simulink model "ASM_Traffic_V2X_Complete_Model_2"  (R2019a)
settings: Solver=ode1  StartTime=SIM.tstart.v  StopTime=Inf  FixedStep=SIM.StepSize.v  RelTol=1e-3
PostLoadFcn:
  | if any(exist('dsrtsu_mdlpostloadfcn', 'file') ~= 0), dsrtsu_mdlpostloadfcn('Execute', bdroot); end
  | try, asm_mdl_postloadfcn(bdroot, 'UpdateModel', 2200); catch, disp(lasterr); end,
undefined symbols (not defined in the file): _SensorPnts_1, _SensorPnts_13, _SensorPnts_17, _SensorPnts_21, _SensorPnts_25, _SensorPnts_29, _SensorPnts_33, _SensorPnts_37, _SensorPnts_41, _SensorPnts_45, _SensorPnts_49, _SensorPnts_5, _SensorPnts_53, _SensorPnts_57, _SensorPnts_9, _to_, CPT, G5A, ITS, MDL, rad, s_to_rpm, SIM
libraries: simulink x169, ASM_VehicleDynamics_lib x126, ASM_Traffic_lib x83, ASM_Utils_lib x49, mdbs x45, ASM_Environment_lib x17, dspindex x12, dsaV2xLibraryAux x10, dsmpblib x6, dsaV2xAsn1Library x4, dsaV2xLibrary x4, ASM_BrakeHydraulics_lib x4
(part 24 of 36)

== system ASM_Traffic_V2X_Complete_Model_2/MDL/Environment/EnvironmentInterface_In/VehicleMovement/Mapping_Vel/YawRate_Vehicle_CoG[deg|s]1 ==
  In1 : Inport
  Out1 : Outport
  wires:
  In1/1 -> Out1/1

== system ASM_Traffic_V2X_Complete_Model_2/MDL/Environment/EnvironmentInterface_In/VehicleMovement/Mapping_Vel/v_x_Vehicle_CoG[km|h]1 ==
  In1 : Inport
  Out1 : Outport
  wires:
  In1/1 -> Out1/1

== system ASM_Traffic_V2X_Complete_Model_2/MDL/Environment/EnvironmentInterface_In/VehicleMovement/Mapping_Vel/v_y_Vehicle_CoG[km|h]1 ==
  In1 : Inport
  Out1 : Outport
  wires:
  In1/1 -> Out1/1

== system ASM_Traffic_V2X_Complete_Model_2/MDL/Environment/Maneuver/ExternalSegmentEnd/Dist_Front_Min/Replace_NoObjectFound1 ==
  In1 : Inport
  Far_away : Constant  Value=1000
  No_Hinderance : Constant  Value=0
  Relational Operator : RelationalOperator  Operator=<=  RndMeth=Nearest  InputSameDT=on
  Switch : Switch  Threshold=1  InputSameDT=on
  Out1 : Outport
  wires:
  No_Hinderance/1 -> Relational Operator/2
  Relational Operator/1 -> Switch/2
  Far_away/1 -> Switch/1
  In1/1 -> Relational Operator/1, Switch/3
  Switch/1 -> Out1/1

== system ASM_Traffic_V2X_Complete_Model_2/MDL/Environment/Maneuver/ExternalSegmentEnd/Dist_Rear_Min/Replace_NoObjectFound1 ==
  In1 : Inport
  Far_away : Constant  Value=1000
  No_Hinderance : Constant  Value=0
  Relational Operator : RelationalOperator  Operator=<=  RndMeth=Nearest  InputSameDT=on
  Switch : Switch  Threshold=1  InputSameDT=on
  Out1 : Outport
  wires:
  Switch/1 -> Out1/1
  In1/1 -> Switch/3, Relational Operator/1
  Far_away/1 -> Switch/1
  Relational Operator/1 -> Switch/2
  No_Hinderance/1 -> Relational Operator/2

== system ASM_Traffic_V2X_Complete_Model_2/MDL/Environment/Maneuver/ExternalSegmentEnd/SegmentEndTrigger/Fishhook ==
  RollRate_Threshold[deg|s] : Inport
  RollRate_Vehicle_CoG[deg|s] : Inport  Port=2
  Abs : Abs  SaturateOnIntegerOverflow=on
  Fcn_1 : Fcn  Expr=(u[1]>=0.0)*(u[2]<0.0)
  Fcn_2 : Fcn  Expr=(u[1]>0.0)
  Memory1 : Memory
  Memory2 : Memory
  Mux : Mux  Inputs=2
  Product : Product  RndMeth=Zero
  Sum : Sum  Inputs=|-+  SaturateOnIntegerOverflow=on
  SegmentEnd_Fishhook : Outport
  wires:
  Memory1/1 -> Mux/1
  Mux/1 -> Fcn_1/1
  Sum/1 -> Memory1/1, Mux/2
  Abs/1 -> Sum/2
  RollRate_Threshold[deg|s]/1 -> Sum/1, Memory2/1
  RollRate_Vehicle_CoG[deg|s]/1 -> Abs/1
  Memory2/1 -> Fcn_2/1
  Fcn_2/1 -> Product/1
  Fcn_1/1 -> Product/2
  Product/1 -> SegmentEnd_Fishhook/1

== system ASM_Traffic_V2X_Complete_Model_2/MDL/Environment/Maneuver/ExternalSegmentEnd/SegmentEndTrigger/SaturateAndRound ==
  In : Inport
  Max : Inport  Port=2
  Const_zero : Constant  Value=0
  Data Type Conversion : DataTypeConversion
  Log_and : Logic  Inputs=3  AllPortsSameDT=off  OutDataTypeStr=boolean
  Product : Product  RndMeth=Zero
  RelOp1 : RelationalOperator  Operator===  OutDataTypeStr=boolean  RndMeth=Nearest
  RelOp2 : RelationalOperator  Operator=<=  OutDataTypeStr=boolean  RndMeth=Nearest
  RelOp3 : RelationalOperator  OutDataTypeStr=boolean  RndMeth=Nearest
  Round : Rounding  Operator=round
  ExternalSegmentEnd_Mode[] : Outport
  wires:
  In/1 -> Product/1, RelOp2/1, RelOp3/1, RelOp1/2, Round/1
  Round/1 -> RelOp1/1
  RelOp1/1 -> Log_and/1
  Log_and/1 -> Data Type Conversion/1
  Data Type Conversion/1 -> Product/2
  Const_zero/1 -> RelOp3/2
  RelOp3/1 -> Log_and/2
  RelOp2/1 -> Log_and/3
  Product/1 -> ExternalSegmentEnd_Mode[]/1
  Max/1 -> RelOp2/2

== system ASM_Traffic_V2X_Complete_Model_2/MDL/Environment/Traffic/FellowMovement/Customize_UserSignals/Label ==
  In1 : Inport
  Out1 : Outport
  wires:
  In1/1 -> Out1/1

== system ASM_Traffic_V2X_Complete_Model_2/MDL/Environment/Traffic/FellowMovement/Customize_UserSignals/Label1 ==
  In1 : Inport
  Out1 : Outport
  wires:
  In1/1 -> Out1/1

== system ASM_Traffic_V2X_Complete_Model_2/MDL/Environment/Traffic/FellowMovement/Customize_UserSignals/Label10 ==
  In1 : Inport
  Out1 : Outport
  wires:
  In1/1 -> Out1/1

== system ASM_Traffic_V2X_Complete_Model_2/MDL/Environment/Traffic/FellowMovement/Customize_UserSignals/Label11 ==
  In1 : Inport
  Out1 : Outport
  wires:
  In1/1 -> Out1/1

== system ASM_Traffic_V2X_Complete_Model_2/MDL/Environment/Traffic/FellowMovement/Customize_UserSignals/Label12 ==
  In1 : Inport
  Out1 : Outport
  wires:
  In1/1 -> Out1/1

== system ASM_Traffic_V2X_Complete_Model_2/MDL/Environment/Traffic/FellowMovement/Customize_UserSignals/Label13 ==
  In1 : Inport
  Out1 : Outport
  wires:
  In1/1 -> Out1/1

== system ASM_Traffic_V2X_Complete_Model_2/MDL/Environment/Traffic/FellowMovement/Customize_UserSignals/Label14 ==
  In1 : Inport
  Out1 : Outport
  wires:
  In1/1 -> Out1/1

== system ASM_Traffic_V2X_Complete_Model_2/MDL/Environment/Traffic/FellowMovement/Customize_UserSignals/Label2 ==
  In1 : Inport
  Out1 : Outport
  wires:
  In1/1 -> Out1/1

== system ASM_Traffic_V2X_Complete_Model_2/MDL/Environment/Traffic/FellowMovement/Customize_UserSignals/Label3 ==
  In1 : Inport
  Out1 : Outport
  wires:
  In1/1 -> Out1/1

== system ASM_Traffic_V2X_Complete_Model_2/MDL/Environment/Traffic/FellowMovement/Customize_UserSignals/Label4 ==
  In1 : Inport
  Out1 : Outport
  wires:
  In1/1 -> Out1/1

== system ASM_Traffic_V2X_Complete_Model_2/MDL/Environment/Traffic/FellowMovement/Customize_UserSignals/Label5 ==
  In1 : Inport
  Out1 : Outport
  wires:
  In1/1 -> Out1/1

== system ASM_Traffic_V2X_Complete_Model_2/MDL/Environment/Traffic/FellowMovement/Customize_UserSignals/Label6 ==
  In1 : Inport
  Out1 : Outport
  wires:
  In1/1 -> Out1/1

== system ASM_Traffic_V2X_Complete_Model_2/MDL/Environment/Traffic/FellowMovement/Customize_UserSignals/Label7 ==
  In1 : Inport
  Out1 : Outport
  wires:
  In1/1 -> Out1/1

== system ASM_Traffic_V2X_Complete_Model_2/MDL/Environment/Traffic/FellowMovement/Customize_UserSignals/Label8 ==
  In1 : Inport
  Out1 : Outport
  wires:
  In1/1 -> Out1/1

== system ASM_Traffic_V2X_Complete_Model_2/MDL/Environment/Traffic/FellowMovement/Customize_UserSignals/Label9 ==
  In1 : Inport
  Out1 : Outport
  wires:
  In1/1 -> Out1/1

== system ASM_Traffic_V2X_Complete_Model_2/MDL/Environment/Traffic/FellowMovement/LabelUserSignals/UserSignals_ ==
  UserSignals : Inport
  Demux : Demux  Outputs=5
  User1[] : Outport
  User2[] : Outport  Port=2
  User3[] : Outport  Port=3
  User4[] : Outport  Port=4
  User5[] : Outport  Port=5
  wires:
  Demux/5 -> User5[]/1
  Demux/4 -> User4[]/1
  UserSignals/1 -> Demux/1
  Demux/1 -> User1[]/1
  Demux/2 -> User2[]/1
  Demux/3 -> User3[]/1

== system ASM_Traffic_V2X_Complete_Model_2/MDL/Environment/Traffic/FellowMovement/LabelUserSignals_Fellows/UserSignals_ ==
  UserSignals : Inport
  Demux : Demux  Outputs=15
  UserSignals_Fellow1[] : Outport
  UserSignals_Fellow2[] : Outport  Port=2
  UserSignals_Fellow3[] : Outport  Port=3
  UserSignals_Fellow4[] : Outport  Port=4
  UserSignals_Fellow5[] : Outport  Port=5
  UserSignals_Fellow6[] : Outport  Port=6
  UserSignals_Fellow7[] : Outport  Port=7
  UserSignals_Fellow8[] : Outport  Port=8
  UserSignals_Fellow9[] : Outport  Port=9
  UserSignals_Fellow10[] : Outport  Port=10
  UserSignals_Fellow11[] : Outport  Port=11
  UserSignals_Fellow12[] : Outport  Port=12
  UserSignals_Fellow13[] : Outport  Port=13
  UserSignals_Fellow14[] : Outport  Port=14
  UserSignals_Fellow15[] : Outport  Port=15
  wires:
  Demux/15 -> UserSignals_Fellow15[]/1  "User1[]"
  Demux/14 -> UserSignals_Fellow14[]/1  "User2[]"
  Demux/13 -> UserSignals_Fellow13[]/1  "User1[]"
  Demux/12 -> UserSignals_Fellow12[]/1  "User2[]"
  Demux/11 -> UserSignals_Fellow11[]/1  "User1[]"
  Demux/10 -> UserSignals_Fellow10[]/1  "User2[]"
  Demux/9 -> UserSignals_Fellow9[]/1  "User1[]"
  Demux/8 -> UserSignals_Fellow8[]/1  "User2[]"
  Demux/7 -> UserSignals_Fellow7[]/1  "User1[]"
  Demux/6 -> UserSignals_Fellow6[]/1  "User2[]"
  Demux/5 -> UserSignals_Fellow5[]/1  "User1[]"
  Demux/4 -> UserSignals_Fellow4[]/1  "User2[]"
  Demux/3 -> UserSignals_Fellow3[]/1  "User1[]"
  Demux/2 -> UserSignals_Fellow2[]/1  "User2[]"
  Demux/1 -> UserSignals_Fellow1[]/1  "User1[]"
  UserSignals/1 -> Demux/1

== system ASM_Traffic_V2X_Complete_Model_2/MDL/Environment/Traffic/FellowMovement/Sw_SpeedLimit_Enable/SpeedLimit_RateLimiter ==
  In : Inport
  Gain : Gain  Gain=-1
  Multiport Switch : MultiPortSwitch  DataPortOrder=Zero-based contiguous  Inputs=2  DiagnosticForDefault=Warning  zeroidx=on
  Rate Limiter Dynamic : simulink/Discontinuities/Rate Limiter Dynamic
      settings: SourceProductName=Simulink
  RateLimit_ActivateThreshold[km|h] : simulink/Logic and Bit Operations/Compare To Constant  relop=>  const=200  OutDataTypeStr=uint8
  SpeedLimit_ChangeRate[km|h|s] : Constant  Value=20.0*ones(MDL.Traffic.MaxNumFellows.v,1)
  Unit Delay : UnitDelay  SampleTime=-1
  off : Constant  Value=1e8*ones(MDL.Traffic.MaxNumFellows.v,1)
  Out : Outport
  wires:
  Unit Delay/1 -> Rate Limiter Dynamic/1, Gain/1
  Rate Limiter Dynamic/1 -> Out/1
  In/1 -> RateLimit_ActivateThreshold[km|h]/1, Rate Limiter Dynamic/2
  Gain/1 -> Rate Limiter Dynamic/3
  Multiport Switch/1 -> Unit Delay/1
  SpeedLimit_ChangeRate[km|h|s]/1 -> Multiport Switch/2
  off/1 -> Multiport Switch/3
  RateLimit_ActivateThreshold[km|h]/1 -> Multiport Switch/1

== system ASM_Traffic_V2X_Complete_Model_2/MDL/Environment/Traffic/Sensors/Collision_Sensor/ASMSignalCollector ==
  Bus Creator3 : BusCreator  Inputs=1
  tag scope: ASMBUS_Environment_Traffic_Sensors_Collision_Sensor=global
  wires:
  [ASMBUS_Traf_Sensors_Collision_Sensor_1] -> Bus Creator3/1  "Collision_Sensor_1"
  Bus Creator3/1 -> [ASMBUS_Environment_Traffic_Sensors_Collision_Sensor]  "Collision_Sensor"

== system ASM_Traffic_V2X_Complete_Model_2/MDL/Environment/Traffic/Sensors/Collision_Sensor/Enable_Collision_Sensor ==
  Enable_In[0Off|1On] : Inport
  Constant : Constant  Value=0.5  SampleTime=-1
  Constant1 : Constant  SampleTime=-1
  Constant2 : Constant  Value=0  SampleTime=-1
  Enable_Sensor : Gain
  Multiport Switch : MultiPortSwitch  DataPortOrder=Zero-based contiguous  Inputs=2  zeroidx=on
  Relational Operator : RelationalOperator  Operator=>  OutDataTypeStr=boolean  RndMeth=Nearest
  Enable_Out[0Off|1On] : Outport
  wires:
  Enable_In[0Off|1On]/1 -> Enable_Sensor/1
  Enable_Sensor/1 -> Relational Operator/1
  Relational Operator/1 -> Multiport Switch/1
  Multiport Switch/1 -> Enable_Out[0Off|1On]/1
  Constant/1 -> Relational Operator/2
  Constant1/1 -> Multiport Switch/3
  Constant2/1 -> Multiport Switch/2

== system ASM_Traffic_V2X_Complete_Model_2/MDL/Environment/Traffic/Sensors/Custom_Sensor/ASMSignalBus_Mapping ==
  ScopezoneData : Inport
  ObjectData : Inport  Port=2
  Bus Creator : BusCreator  Inputs=5
  Bus Creator1 : BusCreator  Inputs=2
  Bus Selector6 : BusSelector  OutputSignals=Info,SensorOutput.Object1,SensorOutput.Object2,SensorOutput.Object3,SensorOutput.Object4,SensorOutput.Object5
  Bus Selector8 : BusSelector  OutputSignals=Info,SensorOutput.Object1,SensorOutput.Object2,SensorOutput.Object3,SensorOutput.Object4,SensorOutput.Object5
  Combine1 : Subsystem
  Combine2 : Subsystem
  Combine3 : Subsystem
  Combine4 : Subsystem
  Combine5 : Subsystem
  CombineInfo : Subsystem
  ASMSignalBus : Outport
  wires:
  CombineInfo/1(Combined_Out) -> Bus Creator1/1  "Info"
  Bus Selector8/1 -> CombineInfo/2(Values_In)  "<Info>"
  Bus Selector6/1 -> CombineInfo/1(Scopezone_In)  "<Info>"
  Bus Creator1/1 -> ASMSignalBus/1
  Bus Selector6/2 -> Combine1/1(Scopezone_In)  "<Object1>"
  Bus Selector8/2 -> Combine1/2(Values_In)  "<Object1>"
  ScopezoneData/1 -> Bus Selector6/1
  ObjectData/1 -> Bus Selector8/1
  Combine1/1(Combined_Out) -> Bus Creator/1  "Object1"
  Combine2/1(Combined_Out) -> Bus Creator/2  "Object2"
  Bus Selector6/3 -> Combine2/1(Scopezone_In)  "<Object2>"
  Bus Selector8/3 -> Combine2/2(Values_In)  "<Object2>"
  Combine3/1(Combined_Out) -> Bus Creator/3  "Object3"
  Bus Selector6/4 -> Combine3/1(Scopezone_In)  "<Object3>"
  Bus Selector8/4 -> Combine3/2(Values_In)  "<Object3>"
  Combine4/1(Combined_Out) -> Bus Creator/4  "Object4"
  Bus Selector6/5 -> Combine4/1(Scopezone_In)  "<Object4>"
  Bus Selector8/5 -> Combine4/2(Values_In)  "<Object4>"
  Combine5/1(Combined_Out) -> Bus Creator/5  "Object5"
  Bus Selector8/6 -> Combine5/2(Values_In)  "<Object5>"
  Bus Selector6/6 -> Combine5/1(Scopezone_In)  "<Object5>"
  Bus Creator/1 -> Bus Creator1/2  "SensorOutput"

== system ASM_Traffic_V2X_Complete_Model_2/MDL/Environment/Traffic/Sensors/Custom_Sensor/ASMSignalCollector ==
  Bus Creator1 : BusCreator  Inputs=3
  Bus Creator3 : BusCreator  Inputs=1
  Bus Selector : BusSelector  OutputSignals=Info,SensorOutput
  tag scope: ASMBUS_Environment_Traffic_Sensors_Custom_Sensor=global
  wires:
  [ASMBUS_Environment_Traffic_Sensors_Custom_Sensor_1_Parameters] -> Bus Creator1/3  "Parameters"
  Bus Selector/2 -> Bus Creator1/2  "<SensorOutput>"
  Bus Selector/1 -> Bus Creator1/1  "<Info>"
  [ASMBUS_Environment_Traffic_Sensors_Custom_Sensor_1] -> Bus Selector/1
  Bus Creator3/1 -> [ASMBUS_Environment_Traffic_Sensors_Custom_Sensor]  "Custom_Sensor"
  Bus Creator1/1 -> Bus Creator3/1  "Sensor_Front_1"

== system ASM_Traffic_V2X_Complete_Model_2/MDL/Environment/Traffic/Sensors/Custom_Sensor/Enable_Custom_Sensor ==
  Enable_In[0Off|1On] : Inport
  Constant : Constant  Value=0.5  SampleTime=-1
  Constant1 : Constant  SampleTime=-1
  Constant2 : Constant  Value=0  SampleTime=-1
  Enable_Sensor : Gain
  Multiport Switch : MultiPortSwitch  DataPortOrder=Zero-based contiguous  Inputs=2  zeroidx=on
  Relational Operator : RelationalOperator  Operator=>  OutDataTypeStr=boolean  RndMeth=Nearest
  Enable_Out[0Off|1On] : Outport
  wires:
  Constant2/1 -> Multiport Switch/2
  Constant1/1 -> Multiport Switch/3
  Constant/1 -> Relational Operator/2
  Multiport Switch/1 -> Enable_Out[0Off|1On]/1
  Relational Operator/1 -> Multiport Switch/1
  Enable_Sensor/1 -> Relational Operator/1
  Enable_In[0Off|1On]/1 -> Enable_Sensor/1

== system ASM_Traffic_V2X_Complete_Model_2/MDL/Environment/Traffic/Sensors/Custom_Sensor/SensorOutput_Mapping ==
  ScopezoneData : Inport
  ObjectData : Inport  Port=2
  Bus Creator : BusCreator  Inputs=5
  Bus Creator1 : BusCreator  Inputs=1
  Bus Selector6 : BusSelector  OutputSignals=SensorOutput.Object1,SensorOutput.Object2,SensorOutput.Object3,SensorOutput.Object4,SensorOutput.Object5
  Bus Selector8 : BusSelector  OutputSignals=SensorOutput.Object1,SensorOutput.Object2,SensorOutput.Object3,SensorOutput.Object4,SensorOutput.Object5
  Combine1 : Subsystem
  Combine2 : Subsystem
  Combine3 : Subsystem
  Combine4 : Subsystem
  Combine5 : Subsystem
  Sensor_Signals : Outport
  wires:
  Bus Creator/1 -> Bus Creator1/1  "SensorOutput"
  Bus Selector6/5 -> Combine5/1(Scopezone_In)  "<Object5>"
  Bus Selector8/5 -> Combine5/2(Values_In)  "<Object5>"
  Combine5/1(Combined_Out) -> Bus Creator/5  "Object5"
  Bus Selector8/4 -> Combine4/2(Values_In)  "<Object4>"
  Bus Selector6/4 -> Combine4/1(Scopezone_In)  "<Object4>"
  Combine4/1(Combined_Out) -> Bus Creator/4  "Object4"
  Bus Selector8/3 -> Combine3/2(Values_In)  "<Object3>"
  Bus Selector6/3 -> Combine3/1(Scopezone_In)  "<Object3>"
  Combine3/1(Combined_Out) -> Bus Creator/3  "Object3"
  Bus Selector8/2 -> Combine2/2(Values_In)  "<Object2>"
  Bus Selector6/2 -> Combine2/1(Scopezone_In)  "<Object2>"
  Combine2/1(Combined_Out) -> Bus Creator/2  "Object2"
  Combine1/1(Combined_Out) -> Bus Creator/1  "Object1"
  ObjectData/1 -> Bus Selector8/1
  ScopezoneData/1 -> Bus Selector6/1
  Bus Selector8/1 -> Combine1/2(Values_In)  "<Object1>"
  Bus Selector6/1 -> Combine1/1(Scopezone_In)  "<Object1>"
  Bus Creator1/1 -> Sensor_Signals/1

== system ASM_Traffic_V2X_Complete_Model_2/MDL/Environment/Traffic/Sensors/Custom_Sensor/TrafficObject_Type ==
  In1 : Inport
  Bus Selector1 : BusSelector  OutputSignals=SensorOutput.Object1.Object_Type[],SensorOutput.Object2.Object_Type[],SensorOutput.Object3.Object_Type[],SensorOutput.Object4.Object_Type[],SensorOutput.Object5.Object_Type[]
  Mux : Mux  Inputs=5
  Out1 : Outport
  wires:
  Mux/1 -> Out1/1
  Bus Selector1/5 -> Mux/5  "<Object_Type[]>"
  Bus Selector1/4 -> Mux/4  "<Object_Type[]>"
  Bus Selector1/3 -> Mux/3  "<Object_Type[]>"
  Bus Selector1/2 -> Mux/2  "<Object_Type[]>"
  Bus Selector1/1 -> Mux/1  "<Object_Type[]>"
  In1/1 -> Bus Selector1/1

== system ASM_Traffic_V2X_Complete_Model_2/MDL/Environment/Traffic/Sensors/Line_Sensor/ASMSignalCollector ==
  note: LineSensor-Output not
      | fed into SignalBus due
      | to large amount of signal data.
  Add{,1..5} (6 alike) : Sum
  Bus Creator1 : BusCreator  Inputs=8
  Bus Creator{2,4..8} (6 alike) : BusCreator  Inputs=3
  Bus Creator3 : BusCreator  Inputs=1
  Bus Selector : BusSelector  OutputSignals=SensorOutput.Info,SensorOutput.Road,SensorOutput.Junction
  Bus Selector1 : BusSelector  OutputSignals=Road_Lanes.Pos_x_Road_Lanes_CoorSys_E[m],Road_Lanes.Pos_y_Road_Lanes_CoorSys_E[m],Road_Lanes.Pos_z_Road_Lanes_CoorSys_E[m]
  Bus Selector2 : BusSelector  OutputSignals=Junction_Borders.Pos_x_Junction_Borders_CoorSys_E[m],Junction_Borders.Pos_y_Junction_Borders_CoorSys_E[m],Junction_Borders.Pos_z_Junction_Borders_CoorSys_E[m]
  Bus Selector3 : BusSelector  OutputSignals=Road_Shape_Lines.Pos_x_Road_Shape_Lines_CoorSys_E[m],Road_Shape_Lines.Pos_y_Road_Shape_Lines_CoorSys_E[m],Road_Shape_Lines.Pos_z_Road_Shape_Lines_CoorSys_E[m]
  Bus Selector4 : BusSelector  OutputSignals=Road_Shape_ContObj.Pos_x_Road_Shape_ContObj_CoorSys_E[m],Road_Shape_ContObj.Pos_y_Road_Shape_ContObj_CoorSys_E[m],Road_Shape_ContObj.Pos_z_Road_Shape_ContObj_CoorSys_E[m]
  Bus Selector5 : BusSelector  OutputSignals=Junction_Shape_Lines.Pos_x_Junction_Shape_Lines_CoorSys_E[m],Junction_Shape_Lines.Pos_y_Junction_Shape_Lines_CoorSys_E[m],Junction_Shape_Lines.Pos_z_Junction_Shape_Lines_CoorSys_E[m]
  Bus Selector6 : BusSelector  OutputSignals=Junction_Shape_ContObj.Pos_x_Junction_Shape_ContObj_CoorSys_E[m],Junction_Shape_ContObj.Pos_y_Junction_Shape_ContObj_CoorSys_E[m],Junction_Shape_ContObj.Pos_z_Junction_Shape_ContObj_CoorSys_E[m]
  Dummy : Constant  Value=0
  Idx_Vector_Junction_Borders : Constant  Value=1:1:60
  Idx_Vector_Junction_Shape_ContObj : Constant  Value=1:1:60
  Idx_Vector_Junction_Shape_Lines : Constant  Value=1:1:60
  Idx_Vector_Road_Lanes : Constant  Value=1:1:60
  Idx_Vector_Road_Shape_ContObj : Constant  Value=1:1:60
  Idx_Vector_Road_Shape_Lines : Constant  Value=1:1:60
  Saturation : Saturate  UpperLimit=MDL.Traffic.Sensors.LineSensor.Const_Road_Lane_Output_Dimension.v  LowerLimit=1
  Saturation1 : Saturate  UpperLimit=MDL.Traffic.Sensors.LineSensor.Const_Road_Shape_Line_Output_Dimension.v  LowerLimit=1
  Saturation2 : Saturate  UpperLimit=MDL.Traffic.Sensors.LineSensor.Const_Road_Shape_ContObj_Output_Dimension.v  LowerLimit=1
  Saturation3 : Saturate  UpperLimit=MDL.Traffic.Sensors.LineSensor.Const_Junction_Border_Output_Dimension.v  LowerLimit=1
  Saturation4 : Saturate  UpperLimit=MDL.Traffic.Sensors.LineSensor.Const_Junction_Border_Output_Dimension.v  LowerLimit=1
  Saturation5 : Saturate  UpperLimit=MDL.Traffic.Sensors.LineSensor.Const_Junction_Border_Output_Dimension.v  LowerLimit=1
  Selector1 : Selector  InputPortWidth=MDL.Traffic.Sensors.LineSensor.Const_Road_Lane_Output_Dimension.v  IndexOptions=Index vector (port)  Indices=1  OutputSizes=36
  Selector10 : Selector  InputPortWidth=MDL.Traffic.Sensors.LineSensor.Const_Road_Shape_ContObj_Output_Dimension.v  IndexOptions=Index vector (port)  Indices=1  OutputSizes=36
  Selector11 : Selector  InputPortWidth=MDL.Traffic.Sensors.LineSensor.Const_Road_Shape_ContObj_Output_Dimension.v  IndexOptions=Index vector (port)  Indices=1  OutputSizes=36
  Selector12 : Selector  InputPortWidth=MDL.Traffic.Sensors.LineSensor.Const_Road_Shape_ContObj_Output_Dimension.v  IndexOptions=Index vector (port)  Indices=1  OutputSizes=36
  Selector13 : Selector  InputPortWidth=MDL.Traffic.Sensors.LineSensor.Const_Junction_Shape_Line_Output_Dimension.v  IndexOptions=Index vector (port)  Indices=1  OutputSizes=36
  Selector14 : Selector  InputPortWidth=MDL.Traffic.Sensors.LineSensor.Const_Junction_Shape_Line_Output_Dimension.v  IndexOptions=Index vector (port)  Indices=1  OutputSizes=36
  Selector15 : Selector  InputPortWidth=MDL.Traffic.Sensors.LineSensor.Const_Junction_Shape_Line_Output_Dimension.v  IndexOptions=Index vector (port)  Indices=1  OutputSizes=36
  Selector16 : Selector  InputPortWidth=MDL.Traffic.Sensors.LineSensor.Const_Junction_Shape_ContObj_Output_Dimension.v  IndexOptions=Index vector (port)  Indices=1  OutputSizes=36
  Selector17 : Selector  InputPortWidth=MDL.Traffic.Sensors.LineSensor.Const_Junction_Shape_ContObj_Output_Dimension.v  IndexOptions=Index vector (port)  Indices=1  OutputSizes=36
  Selector18 : Selector  InputPortWidth=MDL.Traffic.Sensors.LineSensor.Const_Junction_Shape_ContObj_Output_Dimension.v  IndexOptions=Index vector (port)  Indices=1  OutputSizes=36
  Selector2 : Selector  InputPortWidth=MDL.Traffic.Sensors.LineSensor.Const_Road_Lane_Output_Dimension.v  IndexOptions=Index vector (port)  Indices=1  OutputSizes=36
  Selector3 : Selector  InputPortWidth=MDL.Traffic.Sensors.LineSensor.Const_Road_Lane_Output_Dimension.v  IndexOptions=Index vector (port)  Indices=1  OutputSizes=36
  Selector4 : Selector  InputPortWidth=MDL.Traffic.Sensors.LineSensor.Const_Junction_Border_Output_Dimension.v  IndexOptions=Index vector (port)  Indices=1  OutputSizes=36
  Selector5 : Selector  InputPortWidth=MDL.Traffic.Sensors.LineSensor.Const_Junction_Border_Output_Dimension.v  IndexOptions=Index vector (port)  Indices=1  OutputSizes=36
  Selector6 : Selector  InputPortWidth=MDL.Traffic.Sensors.LineSensor.Const_Junction_Border_Output_Dimension.v  IndexOptions=Index vector (port)  Indices=1  OutputSizes=36
  Selector7 : Selector  InputPortWidth=MDL.Traffic.Sensors.LineSensor.Const_Road_Shape_Line_Output_Dimension.v  IndexOptions=Index vector (port)  Indices=1  OutputSizes=36
  Selector8 : Selector  InputPortWidth=MDL.Traffic.Sensors.LineSensor.Const_Road_Shape_Line_Output_Dimension.v  IndexOptions=Index vector (port)  Indices=1  OutputSizes=36
  Selector9 : Selector  InputPortWidth=MDL.Traffic.Sensors.LineSensor.Const_Road_Shape_Line_Output_Dimension.v  IndexOptions=Index vector (port)  Indices=1  OutputSizes=36
  Signal Specification{,1..5} (6 alike) : SignalSpecification  Dimensions=60
  z_Offset[m] : Constant  Value=0.1
  tag scope: ASMBUS_Environment_Traffic_Sensors_Line_Sensor=global
  wires:
  Dummy/1 -> Bus Creator1/8  "Dummy_SensorOutput"
  Saturation5/1 -> Signal Specification5/1
  Idx_Vector_Junction_Shape_ContObj/1 -> Saturation5/1
  Signal Specification5/1 -> Selector18/2, Selector16/2, Selector17/2
  Bus Creator8/1 -> Bus Creator1/7  "Pos_Junction_Shape_ContObj_Animation_CoorSys_E"
  Add4/1 -> Bus Creator8/3  "Pos_z_Junction_Shape_ContObj_Animation_CoorSys_E"
  Selector17/1 -> Add4/1
  Selector16/1 -> Bus Creator8/2  "Pos_y_Junction_Shape_ContObj_Animation_CoorSys_E"
  Selector18/1 -> Bus Creator8/1  "Pos_x_Junction_Shape_ContObj_Animation_CoorSys_E"
  Bus Selector6/3 -> Selector17/1  "<Pos_z_Junction_Shape_ContObj_CoorSys_E[m]>"
  Bus Selector6/2 -> Selector16/1  "<Pos_y_Junction_Shape_ContObj_CoorSys_E[m]>"
  Bus Selector6/1 -> Selector18/1  "<Pos_x_Junction_Shape_ContObj_CoorSys_E[m]>"
  Bus Selector/3 -> Bus Selector2/1, Bus Selector5/1, Bus Selector6/1  "<Junction>"
  Saturation4/1 -> Signal Specification4/1
  Idx_Vector_Junction_Shape_Lines/1 -> Saturation4/1
  Signal Specification4/1 -> Selector15/2, Selector13/2, Selector14/2
  Bus Creator7/1 -> Bus Creator1/6  "Pos_Junction_Shape_Line_Animation_CoorSys_E"
  Add5/1 -> Bus Creator7/3  "Pos_z_Junction_Shape_Line_Animation_CoorSys_E"
  Selector14/1 -> Add5/1
  Selector13/1 -> Bus Creator7/2  "Pos_y_Junction_Shape_Line_Animation_CoorSys_E"
  Selector15/1 -> Bus Creator7/1  "Pos_x_Junction_Shape_Line_Animation_CoorSys_E"
  Bus Selector5/3 -> Selector14/1  "<Pos_z_Junction_Shape_Lines_CoorSys_E[m]>"
  Bus Selector5/2 -> Selector13/1  "<Pos_y_Junction_Shape_Lines_CoorSys_E[m]>"
  Bus Selector5/1 -> Selector15/1  "<Pos_x_Junction_Shape_Lines_CoorSys_E[m]>"
  Signal Specification3/1 -> Selector6/2, Selector4/2, Selector5/2
  Saturation3/1 -> Signal Specification3/1
  Idx_Vector_Junction_Borders/1 -> Saturation3/1
  Signal Specification2/1 -> Selector12/2, Selector10/2, Selector11/2
  Saturation2/1 -> Signal Specification2/1
  Idx_Vector_Road_Shape_ContObj/1 -> Saturation2/1
  Signal Specification1/1 -> Selector9/2, Selector7/2, Selector8/2
  Saturation1/1 -> Signal Specification1/1
  Idx_Vector_Road_Shape_Lines/1 -> Saturation1/1
  Signal Specification/1 -> Selector2/2, Selector1/2, Selector3/2
  Bus Creator4/1 -> Bus Creator1/5  "Pos_Junction_Border_Animation_CoorSys_E"
  Bus Creator6/1 -> Bus Creator1/4  "Pos_Road_Shape_ContObj_Animation_CoorSys_E"
  Bus Creator5/1 -> Bus Creator1/3  "Pos_Road_Shape_Line_Animation_CoorSys_E"
  Add2/1 -> Bus Creator6/3  "Pos_z_Road_Shape_ContObj_Animation_CoorSys_E"
  Selector11/1 -> Add2/1
  Selector10/1 -> Bus Creator6/2  "Pos_y_Road_Shape_ContObj_Animation_CoorSys_E"
  Selector12/1 -> Bus Creator6/1  "Pos_x_Road_Shape_ContObj_Animation_CoorSys_E"
  Bus Selector4/3 -> Selector11/1  "<Pos_z_Road_Shape_ContObj_CoorSys_E[m]>"
  Bus Selector4/2 -> Selector10/1  "<Pos_y_Road_Shape_ContObj_CoorSys_E[m]>"
  Bus Selector4/1 -> Selector12/1  "<Pos_x_Road_Shape_ContObj_CoorSys_E[m]>"
  Bus Selector/2 -> Bus Selector1/1, Bus Selector3/1, Bus Selector4/1  "<Road>"
  z_Offset[m]/1 -> Add4/2, Add3/2, Add/2, Add2/2, Add1/2, Add5/2
  Add3/1 -> Bus Creator5/3  "Pos_z_Road_Shape_Line_Animation_CoorSys_E"
  Selector8/1 -> Add3/1
  Selector7/1 -> Bus Creator5/2  "Pos_y_Road_Shape_Line_Animation_CoorSys_E"
  Selector9/1 -> Bus Creator5/1  "Pos_x_Road_Shape_Line_Animation_CoorSys_E"
  Bus Selector3/3 -> Selector8/1  "<Pos_z_Road_Shape_Lines_CoorSys_E[m]>"
  Bus Selector3/2 -> Selector7/1  "<Pos_y_Road_Shape_Lines_CoorSys_E[m]>"
  Bus Selector3/1 -> Selector9/1  "<Pos_x_Road_Shape_Lines_CoorSys_E[m]>"
  Add1/1 -> Bus Creator4/3  "Pos_z_Junction_Border_Animation_CoorSys_E"
  Selector5/1 -> Add1/1
  Selector4/1 -> Bus Creator4/2  "Pos_y_Junction_Border_Animation_CoorSys_E"
  Selector6/1 -> Bus Creator4/1  "Pos_x_Junction_Border_Animation_CoorSys_E"
  Bus Selector2/3 -> Selector5/1  "<Pos_z_Junction_Borders_CoorSys_E[m]>"
  Bus Selector2/2 -> Selector4/1  "<Pos_y_Junction_Borders_CoorSys_E[m]>"
  Bus Selector2/1 -> Selector6/1  "<Pos_x_Junction_Borders_CoorSys_E[m]>"
  Saturation/1 -> Signal Specification/1
  Add/1 -> Bus Creator2/3  "Pos_z_Road_Lane_Animation_CoorSys_E"
  Idx_Vector_Road_Lanes/1 -> Saturation/1
  Bus Creator2/1 -> Bus Creator1/2  "Pos_Road_Lane_Animation_CoorSys_E"
  Selector2/1 -> Add/1
  Selector1/1 -> Bus Creator2/2  "Pos_y_Road_Lane_Animation_CoorSys_E"
  Selector3/1 -> Bus Creator2/1  "Pos_x_Road_Lane_Animation_CoorSys_E"
  Bus Selector1/3 -> Selector2/1  "<Pos_z_Road_Lanes_CoorSys_E[m]>"
  Bus Selector1/2 -> Selector1/1  "<Pos_y_Road_Lanes_CoorSys_E[m]>"
  Bus Selector1/1 -> Selector3/1  "<Pos_x_Road_Lanes_CoorSys_E[m]>"
  Bus Creator1/1 -> Bus Creator3/1  "Line_Sensor_1"
  Bus Selector/1 -> Bus Creator1/1  "<Info>"
  Bus Creator3/1 -> [ASMBUS_Environment_Traffic_Sensors_Line_Sensor]  "Line_Sensor"
  [ASMBUS_Traf_Sensors_Line_Sensor_1] -> Bus Selector/1

== system ASM_Traffic_V2X_Complete_Model_2/MDL/Environment/Traffic/Sensors/Line_Sensor/Enable_Line_Sensor ==
  Enable_In[0Off|1On] : Inport
  Constant : Constant  Value=0.5  SampleTime=-1
  Constant1 : Constant  SampleTime=-1
  Constant2 : Constant  Value=0  SampleTime=-1
  Enable_Sensor : Gain
  Multiport Switch : MultiPortSwitch  DataPortOrder=Zero-based contiguous  Inputs=2  zeroidx=on
  Relational Operator : RelationalOperator  Operator=>  OutDataTypeStr=boolean  RndMeth=Nearest
  Enable_Out[0Off|1On] : Outport
  wires:
  Constant2/1 -> Multiport Switch/2
  Constant1/1 -> Multiport Switch/3
  Constant/1 -> Relational Operator/2
  Multiport Switch/1 -> Enable_Out[0Off|1On]/1
  Relational Operator/1 -> Multiport Switch/1
  Enable_Sensor/1 -> Relational Operator/1
  Enable_In[0Off|1On]/1 -> Enable_Sensor/1

== system ASM_Traffic_V2X_Complete_Model_2/MDL/Environment/Traffic/Sensors/Object_Sensor_2D/ASMSignalCollector ==
  Bus Creator1 : BusCreator  Inputs=9
  Bus Creator{2..4,6..9} (7 alike) : BusCreator  Inputs=5
  Bus Selector{,1,3..7} (7 alike) : BusSelector  OutputSignals=SensorIndex,SensorStatus,SensorOutput
  tag scope: ASMBUS_Environment_Traffic_Sensors_Object_Sensor_2D=global
  wires:
  Bus Selector1/3 -> Bus Creator4/4  "<SensorOutput>"
  Bus Selector1/2 -> Bus Creator4/3  "<SensorStatus>"
  Bus Selector1/1 -> Bus Creator4/2  "<SensorIndex>"
  [ASMBUS_Environment_Traffic_2DObjSensor6_Parameter] -> Bus Creator4/1  "Parameters"
  Bus Creator4/1 -> Bus Creator1/8  "Sensor_6_Right"
  [ASMBUS_Environment_Traffic_2DObjSensor6_SensorSignals] -> Bus Selector1/1
  Bus Selector7/3 -> Bus Creator9/4  "<SensorOutput>"
  Bus Selector7/2 -> Bus Creator9/3  "<SensorStatus>"
  Bus Selector7/1 -> Bus Creator9/2  "<SensorIndex>"
  [ASMBUS_Environment_Traffic_2DObjSensor7_Parameter] -> Bus Creator9/1  "Parameters"
  Bus Creator9/1 -> Bus Creator1/9  "Sensor_7_Rear_Right"
  [ASMBUS_Environment_Traffic_2DObjSensor7_SensorSignals] -> Bus Selector7/1
  Bus Selector6/3 -> Bus Creator8/4  "<SensorOutput>"
  Bus Selector6/2 -> Bus Creator8/3  "<SensorStatus>"
  Bus Selector6/1 -> Bus Creator8/2  "<SensorIndex>"
  [ASMBUS_Environment_Traffic_2DObjSensor5_Parameter] -> Bus Creator8/1  "Parameters"
  Bus Creator8/1 -> Bus Creator1/7  "Sensor_5_Front_Right"
  [ASMBUS_Environment_Traffic_2DObjSensor5_SensorSignals] -> Bus Selector6/1
  Bus Selector5/3 -> Bus Creator7/4  "<SensorOutput>"
  Bus Selector5/2 -> Bus Creator7/3  "<SensorStatus>"
  Bus Selector5/1 -> Bus Creator7/2  "<SensorIndex>"
  [ASMBUS_Environment_Traffic_2DObjSensor4_Parameter] -> Bus Creator7/1  "Parameters"
  Bus Creator7/1 -> Bus Creator1/6  "Sensor_4_Rear_Left"
  [ASMBUS_Environment_Traffic_2DObjSensor4_SensorSignals] -> Bus Selector5/1
  Bus Selector4/3 -> Bus Creator6/4  "<SensorOutput>"
  Bus Selector4/2 -> Bus Creator6/3  "<SensorStatus>"
  Bus Selector4/1 -> Bus Creator6/2  "<SensorIndex>"
  [ASMBUS_Environment_Traffic_2DObjSensor3_Parameter] -> Bus Creator6/1  "Parameters"
  Bus Creator6/1 -> Bus Creator1/5  "Sensor_3_Left"
  [ASMBUS_Environment_Traffic_2DObjSensor3_SensorSignals] -> Bus Selector4/1
  Bus Selector3/3 -> Bus Creator3/4  "<SensorOutput>"
  Bus Selector3/2 -> Bus Creator3/3  "<SensorStatus>"
  Bus Selector3/1 -> Bus Creator3/2  "<SensorIndex>"
  [ASMBUS_Environment_Traffic_2DObjSensor2_Parameter] -> Bus Creator3/1  "Parameters"
  Bus Creator3/1 -> Bus Creator1/4  "Sensor_2_Front_Left"
  [ASMBUS_Environment_Traffic_2DObjSensor2_SensorSignals] -> Bus Selector3/1
  Bus Selector/3 -> Bus Creator2/4  "<SensorOutput>"
  Bus Selector/2 -> Bus Creator2/3  "<SensorStatus>"
  Bus Selector/1 -> Bus Creator2/2  "<SensorIndex>"
  [ASMBUS_Environment_Traffic_2DObjSensorCalc_Info] -> Bus Creator4/5, Bus Creator2/5, Bus Creator3/5, Bus Creator6/5, Bus Creator7/5, Bus Creator8/5, Bus Creator9/5  "Info"
  [ASMBUS_Environment_Traffic_SamplePulse_ObjectSensor2D] -> Bus Creator1/1  "Sample_Pulse"
  [ASMBUS_Environment_Traffic_SensorScheduler_ObjectSensor2D] -> Bus Creator1/2  "Sensor_Scheduler"
  [ASMBUS_Environment_Traffic_2DObjSensor1_Parameter] -> Bus Creator2/1  "Parameters"
  Bus Creator2/1 -> Bus Creator1/3  "Sensor_1_Front"
  [ASMBUS_Environment_Traffic_2DObjSensor1_SensorSignals] -> Bus Selector/1
  Bus Creator1/1 -> [ASMBUS_Environment_Traffic_Sensors_Object_Sensor_2D]  "Object_Sensor_2D"

== system ASM_Traffic_V2X_Complete_Model_2/MDL/Environment/Traffic/Sensors/Object_Sensor_2D/Enable_Object_Sensor_2D ==
  Enable_In[0Off|1On] : Inport
  Constant : Constant  Value=0.5  SampleTime=-1
  Constant1 : Constant  SampleTime=-1
  Constant2 : Constant  Value=0  SampleTime=-1
  Enable_Sensor : Gain
  Multiport Switch : MultiPortSwitch  DataPortOrder=Zero-based contiguous  Inputs=2  zeroidx=on
  Relational Operator : RelationalOperator  Operator=>  OutDataTypeStr=boolean  RndMeth=Nearest
  Enable_Out[0Off|1On] : Outport
  wires:
  Constant2/1 -> Multiport Switch/2
  Constant1/1 -> Multiport Switch/3
  Constant/1 -> Relational Operator/2
  Multiport Switch/1 -> Enable_Out[0Off|1On]/1
  Relational Operator/1 -> Multiport Switch/1
  Enable_Sensor/1 -> Relational Operator/1
  Enable_In[0Off|1On]/1 -> Enable_Sensor/1

== system ASM_Traffic_V2X_Complete_Model_2/MDL/Environment/Traffic/Sensors/Object_Sensor_2D/ScheduleAndCalculateSensor ==
  Sensor_Data[] : Inport
  Enable[0Off|1On] : Inport  Port=2
  Fellows_Signals : Inport  Port=3
  VehicleDynamics_Signals : Inport  Port=4
  Objects_Signals : Inport  Port=5
  Road_Signals : Inport  Port=6
  Bus Selector : BusSelector  OutputSignals=VehicleMovement.Positions.Pos_Vehicle_CoorSys_E[x;y;z][m].Pos_Vehicle_CoorSys_E[x;y;z][m],VehicleMovement.Positions.Angle_Vehicle_CoorSys_E[x;y;z][deg].Angle_Vehicle_CoorSys_E[x;y;z][deg]
  Bus Selector2 : BusSelector  OutputSignals=Pos_Fellows_MainPnt_CoorSys_E[x;y;z][m],Angle_Fellows[x;y;z][deg],Flag_FellowUsed[0|1]
  Bus Selector3 : BusSelector  OutputSignals=TrafficObject_Type_Fellows[],TrafficObject_Type_Data[],DiscreteObject_Data[]
  Bus Selector4 : BusSelector  OutputSignals=TrafficObject_Data[]  OutputAsBus=on
  Mux : Mux  Inputs=2
  OBJECT_SENSOR_2D_CALCULATION : ASM_Traffic_lib/Sensors/Object_Sensor_2D/OBJECT_SENSOR_2D_CALCULATION  Const_Sensor_Output_Dimension=MDL.Traffic.Sensors.ObjectSensor2D_Calculation.Const_Sensor_Output_Dimension  ASMProperties=struct('Name','OBJECT_SENSOR_2D_CALCULATION','Version','8.0','Library','ASM_Traffic_lib')  ASMInstanceName=object_sensor_2d_calculation  ASMInstanceID=1
  OBJECT_SENSOR_2D_PARAM_SELECTION : ASM_Traffic_lib/Sensors/Object_Sensor_2D/OBJECT_SENSOR_2D_PARAM_SELECTION  ASMProperties=struct('Name','OBJECT_SENSOR_2D_PARAM_SELECTION','Version','2.0','Library','ASM_Traffic_lib')  ASMInstanceName=object_sensor_2d_param_selection  ASMInstanceID=1
  OBJECT_SENSOR_2D_PARAM_VECTORIZATION : ASM_Traffic_lib/Sensors/Object_Sensor_2D/OBJECT_SENSOR_2D_PARAM_VECTORIZATION  ASMProperties=struct('Name','OBJECT_SENSOR_2D_PARAM_VECTORIZATION','Version','3.0','Library','ASM_Traffic_lib')  ASMInstanceName=object_sensor_2d_param_vectorization  ASMInstanceID=1
  SAMPLE_PULSE : ASM_Traffic_lib/Sensors/Scheduling/SAMPLE_PULSE  Tag=ASM_SUBCOMPONENT  Sw_SamplePulse=MDL.Traffic.Sensors.SamplePulse_2.Sw_SamplePulse  Const_t_Offs_Pulse=MDL.Traffic.Sensors.SamplePulse_2.Const_t_Offs_Pulse  Const_t_Cycle_Pulse=MDL.Traffic.Sensors.SamplePulse_2.Const_t_Cycle_Pulse  StepSize=SIM.StepSize  ASMProperties=struct('Name','SAMPLE_PULSE','Version','3.0','Library','ASM_Traffic_lib')  ASMInstanceName=sample_pulse  ASMInstanceID=2
      settings: AttributesFormatString=Instance Name: sample_pulse\nInstance ID: 2
  SENSOR_SCHEDULER : ASM_Traffic_lib/Sensors/Scheduling/SENSOR_SCHEDULER  StepSize=SIM.StepSize  ASMProperties=struct('Name','SENSOR_SCHEDULER','Version','4.0','Library','ASM_Traffic_lib')  ASMInstanceName=sensor_scheduler  ASMInstanceID=1
  SampleAndHold : Subsystem  TreatAsAtomicUnit=on
  Terminator{1..5} (5 alike) : Terminator
  SensorMapping_Data[] : Outport
  SensorSignals : Outport  Port=2
  tag scope: ASMBUS_Environment_Traffic_SamplePulse_ObjectSensor2D=global, ASMBUS_Environment_Traffic_SensorScheduler_ObjectSensor2D=global
  wires:
  SampleAndHold/2(Out2) -> OBJECT_SENSOR_2D_CALCULATION/5
  SampleAndHold/1(Out1) -> OBJECT_SENSOR_2D_CALCULATION/4
  SampleAndHold/4(Out4) -> OBJECT_SENSOR_2D_CALCULATION/7
  SampleAndHold/5(Out5) -> OBJECT_SENSOR_2D_CALCULATION/8
  SampleAndHold/3(Out3) -> OBJECT_SENSOR_2D_CALCULATION/6
  Bus Selector3/3 -> OBJECT_SENSOR_2D_CALCULATION/12  "<DiscreteObject_Data[]>"
  Mux/1 -> OBJECT_SENSOR_2D_CALCULATION/1
  SENSOR_SCHEDULER/9 -> Terminator4/1
  SENSOR_SCHEDULER/5 -> OBJECT_SENSOR_2D_CALCULATION/2
  Bus Selector2/3 -> SampleAndHold/5(In5)  "<Flag_FellowUsed[0|1]>"
  SENSOR_SCHEDULER/4 -> Mux/2
  SENSOR_SCHEDULER/3 -> Terminator5/1
  SENSOR_SCHEDULER/2 -> SensorMapping_Data[]/1
  SENSOR_SCHEDULER/6 -> OBJECT_SENSOR_2D_PARAM_SELECTION/1
  Fellows_Signals/1 -> Bus Selector2/1
  VehicleDynamics_Signals/1 -> Bus Selector/1
  Bus Selector4/1 -> OBJECT_SENSOR_2D_CALCULATION/11
  Road_Signals/1 -> Bus Selector4/1
  Bus Selector3/2 -> OBJECT_SENSOR_2D_CALCULATION/10  "<TrafficObject_Type_Data[]>"
  Bus Selector/1 -> SampleAndHold/1(In1)  "<Pos_Vehicle_CoorSys_E[x;y;z][m]>"
  Bus Selector/2 -> SampleAndHold/2(In2)  "<Angle_Vehicle_CoorSys_E[x;y;z][deg]>"
  Bus Selector2/1 -> SampleAndHold/3(In3)  "<Pos_Fellows_MainPnt_CoorSys_E[x;y;z][m]>"
  Bus Selector3/1 -> OBJECT_SENSOR_2D_CALCULATION/9  "<TrafficObject_Type_Fellows[]>"
  Objects_Signals/1 -> Bus Selector3/1
  Bus Selector2/2 -> SampleAndHold/4(In4)  "<Angle_Fellows[x;y;z][deg]>"
  Sensor_Data[]/1 -> OBJECT_SENSOR_2D_PARAM_VECTORIZATION/1
  Enable[0Off|1On]/1 -> SAMPLE_PULSE/1, SENSOR_SCHEDULER/1, Mux/1
  SENSOR_SCHEDULER/7 -> Terminator2/1
  OBJECT_SENSOR_2D_CALCULATION/1 -> Terminator3/1
  OBJECT_SENSOR_2D_PARAM_SELECTION/1 -> OBJECT_SENSOR_2D_CALCULATION/3
  SENSOR_SCHEDULER/8 -> Terminator1/1
  OBJECT_SENSOR_2D_CALCULATION/2 -> SensorSignals/1
  SENSOR_SCHEDULER/1 -> [ASMBUS_Environment_Traffic_SensorScheduler_ObjectSensor2D]
  OBJECT_SENSOR_2D_PARAM_VECTORIZATION/1 -> SENSOR_SCHEDULER/2
  OBJECT_SENSOR_2D_PARAM_VECTORIZATION/2 -> OBJECT_SENSOR_2D_PARAM_SELECTION/2
  SAMPLE_PULSE/2 -> SampleAndHold/Enable
  SAMPLE_PULSE/1 -> [ASMBUS_Environment_Traffic_SamplePulse_ObjectSensor2D]

== system ASM_Traffic_V2X_Complete_Model_2/MDL/Environment/Traffic/Sensors/Object_Sensor_2D/SensorMapping ==
  Enable[0Off|1On] : Inport
  SensorMapping_Data[] : Inport  Port=2
  SensorSignals : Inport  Port=3
  Bus Selector : BusSelector  OutputSignals=Info
  Demux : Demux  Outputs=7
  OBJECT_SENSOR_2D_MAPPING{1..7} (7 alike) : ASM_Traffic_lib/Sensors/Object_Sensor_2D/OBJECT_SENSOR_2D_MAPPING  ASMProperties=struct('Name','OBJECT_SENSOR_2D_MAPPING','Version','1.0','Library','ASM_Traffic_lib')  ASMInstanceName=object_sensor_2d_mapping  ASMInstanceID=1
  Sensor_Signals : Outport
  tag scope: ASMBUS_Environment_Traffic_2DObjSensor1_SensorSignals=global, ASMBUS_Environment_Traffic_2DObjSensor2_SensorSignals=global, ASMBUS_Environment_Traffic_2DObjSensor3_SensorSignals=global, ASMBUS_Environment_Traffic_2DObjSensor4_SensorSignals=global, ASMBUS_Environment_Traffic_2DObjSensor5_SensorSignals=global, ASMBUS_Environment_Traffic_2DObjSensor6_SensorSignals=global, ASMBUS_Environment_Traffic_2DObjSensor7_SensorSignals=global, ASMBUS_Environment_Traffic_2DObjSensorCalc_Info=global
  wires:
  OBJECT_SENSOR_2D_MAPPING7/1 -> [ASMBUS_Environment_Traffic_2DObjSensor7_SensorSignals]
  OBJECT_SENSOR_2D_MAPPING6/1 -> [ASMBUS_Environment_Traffic_2DObjSensor6_SensorSignals]
  OBJECT_SENSOR_2D_MAPPING5/1 -> [ASMBUS_Environment_Traffic_2DObjSensor5_SensorSignals]
  OBJECT_SENSOR_2D_MAPPING4/1 -> [ASMBUS_Environment_Traffic_2DObjSensor4_SensorSignals]
  Demux/7 -> OBJECT_SENSOR_2D_MAPPING7/2
  Demux/6 -> OBJECT_SENSOR_2D_MAPPING6/2
  Demux/5 -> OBJECT_SENSOR_2D_MAPPING5/2
  Demux/4 -> OBJECT_SENSOR_2D_MAPPING4/2
  Enable[0Off|1On]/1 -> OBJECT_SENSOR_2D_MAPPING2/1, OBJECT_SENSOR_2D_MAPPING3/1, OBJECT_SENSOR_2D_MAPPING5/1, OBJECT_SENSOR_2D_MAPPING6/1, OBJECT_SENSOR_2D_MAPPING7/1, OBJECT_SENSOR_2D_MAPPING4/1, OBJECT_SENSOR_2D_MAPPING1/1
  SensorSignals/1 -> Bus Selector/1, OBJECT_SENSOR_2D_MAPPING7/3, OBJECT_SENSOR_2D_MAPPING6/3, OBJECT_SENSOR_2D_MAPPING5/3, OBJECT_SENSOR_2D_MAPPING4/3, OBJECT_SENSOR_2D_MAPPING3/3, OBJECT_SENSOR_2D_MAPPING2/3, OBJECT_SENSOR_2D_MAPPING1/3
  Bus Selector/1 -> [ASMBUS_Environment_Traffic_2DObjSensorCalc_Info]  "<Info>"
  Demux/2 -> OBJECT_SENSOR_2D_MAPPING2/2
  OBJECT_SENSOR_2D_MAPPING3/1 -> [ASMBUS_Environment_Traffic_2DObjSensor3_SensorSignals]
  OBJECT_SENSOR_2D_MAPPING2/1 -> [ASMBUS_Environment_Traffic_2DObjSensor2_SensorSignals]
  SensorMapping_Data[]/1 -> Demux/1
  OBJECT_SENSOR_2D_MAPPING1/1 -> [ASMBUS_Environment_Traffic_2DObjSensor1_SensorSignals], Sensor_Signals/1
  Demux/3 -> OBJECT_SENSOR_2D_MAPPING3/2
  Demux/1 -> OBJECT_SENSOR_2D_MAPPING1/2
